simulink model "AN_Simulink_Model_v1_fil"  (R2019b)
settings: Solver=VariableStepAuto  StartTime=0.0  StopTime=testtime  RelTol=1e-3
InitFcn:
  | AN_InitFcn_Callback
StopFcn:
  | AN_StopFcn_Callback
values from neighbouring files (symbols this model uses):
  tdres = 1/Fs    (= 2.08333333333e-05)    [AN_Set_Model_Parameters.m]
libraries: hdlmdlgenlib x163, simulink x4, fillib x1, dspsrcs4 x1
(part 4 of 5)

== system AN_Simulink_Model_v1_fil/Auditory Nerve Model/C1 Chirp Filter/Get C1 Coefficients/Add7 ==
  In1 : Inport
  In2 : Inport  Port=2
  Add7 : Sum  OutDataTypeStr=single  SampleTime=2.08333333333333e-05  SaturateOnIntegerOverflow=on  InputSameDT=on
  Out1 : Outport
  wires:
  Add7/1 -> Out1/1
  In2/1 -> Add7/2
  In1/1 -> Add7/1

== system AN_Simulink_Model_v1_fil/Auditory Nerve Model/C1 Chirp Filter/Get C1 Coefficients/Add8 ==
  In1 : Inport
  In2 : Inport  Port=2
  Add8 : Sum  OutDataTypeStr=single  SampleTime=2.08333333333333e-05  SaturateOnIntegerOverflow=on  InputSameDT=on
  Out1 : Outport
  wires:
  Add8/1 -> Out1/1
  In2/1 -> Add8/2
  In1/1 -> Add8/1

== system AN_Simulink_Model_v1_fil/Auditory Nerve Model/C1 Chirp Filter/Get C1 Coefficients/Add9 ==
  In1 : Inport
  In2 : Inport  Port=2
  Add9 : Sum  OutDataTypeStr=single  SampleTime=2.08333333333333e-05  SaturateOnIntegerOverflow=on  InputSameDT=on
  Out1 : Outport
  wires:
  Add9/1 -> Out1/1
  In2/1 -> Add9/2
  In1/1 -> Add9/1

== system AN_Simulink_Model_v1_fil/Auditory Nerve Model/C1 Chirp Filter/Get C1 Coefficients/Divide1 ==
  In1 : Inport
  In2 : Inport  Port=2
  Divide1 : Product  Inputs=*/  OutDataTypeStr=single  SampleTime=2.08333333333333e-05  SaturateOnIntegerOverflow=on  RndMeth=Zero
  Out1 : Outport
  wires:
  Divide1/1 -> Out1/1
  In2/1 -> Divide1/2
  In1/1 -> Divide1/1

== system AN_Simulink_Model_v1_fil/Auditory Nerve Model/C1 Chirp Filter/Get C1 Coefficients/Divide10 ==
  In1 : Inport
  In2 : Inport  Port=2
  Divide10 : Product  Inputs=*/  OutDataTypeStr=single  SampleTime=2.08333333333333e-05  SaturateOnIntegerOverflow=on  RndMeth=Zero
  Out1 : Outport
  wires:
  Divide10/1 -> Out1/1
  In2/1 -> Divide10/2
  In1/1 -> Divide10/1

== system AN_Simulink_Model_v1_fil/Auditory Nerve Model/C1 Chirp Filter/Get C1 Coefficients/Divide11 ==
  In1 : Inport
  In2 : Inport  Port=2
  Divide11 : Product  Inputs=*/  OutDataTypeStr=single  SampleTime=2.08333333333333e-05  SaturateOnIntegerOverflow=on  RndMeth=Zero
  Out1 : Outport
  wires:
  Divide11/1 -> Out1/1
  In2/1 -> Divide11/2
  In1/1 -> Divide11/1

== system AN_Simulink_Model_v1_fil/Auditory Nerve Model/C1 Chirp Filter/Get C1 Coefficients/Divide12 ==
  In1 : Inport
  In2 : Inport  Port=2
  Divide12 : Product  Inputs=*/  OutDataTypeStr=single  SampleTime=2.08333333333333e-05  SaturateOnIntegerOverflow=on  RndMeth=Zero
  Out1 : Outport
  wires:
  Divide12/1 -> Out1/1
  In2/1 -> Divide12/2
  In1/1 -> Divide12/1

== system AN_Simulink_Model_v1_fil/Auditory Nerve Model/C1 Chirp Filter/Get C1 Coefficients/Divide13 ==
  In1 : Inport
  In2 : Inport  Port=2
  Divide13 : Product  Inputs=*/  OutDataTypeStr=single  SampleTime=2.08333333333333e-05  SaturateOnIntegerOverflow=on  RndMeth=Zero
  Out1 : Outport
  wires:
  Divide13/1 -> Out1/1
  In2/1 -> Divide13/2
  In1/1 -> Divide13/1

== system AN_Simulink_Model_v1_fil/Auditory Nerve Model/C1 Chirp Filter/Get C1 Coefficients/Divide14 ==
  In1 : Inport
  In2 : Inport  Port=2
  Divide14 : Product  Inputs=*/  OutDataTypeStr=single  SampleTime=2.08333333333333e-05  SaturateOnIntegerOverflow=on  RndMeth=Zero
  Out1 : Outport
  wires:
  Divide14/1 -> Out1/1
  In2/1 -> Divide14/2
  In1/1 -> Divide14/1

== system AN_Simulink_Model_v1_fil/Auditory Nerve Model/C1 Chirp Filter/Get C1 Coefficients/Divide15 ==
  In1 : Inport
  In2 : Inport  Port=2
  Divide15 : Product  Inputs=*/  OutDataTypeStr=single  SampleTime=2.08333333333333e-05  SaturateOnIntegerOverflow=on  RndMeth=Zero
  Out1 : Outport
  wires:
  Divide15/1 -> Out1/1
  In2/1 -> Divide15/2
  In1/1 -> Divide15/1

== system AN_Simulink_Model_v1_fil/Auditory Nerve Model/C1 Chirp Filter/Get C1 Coefficients/Divide16 ==
  In1 : Inport
  In2 : Inport  Port=2
  Divide16 : Product  Inputs=*/  OutDataTypeStr=single  SampleTime=2.08333333333333e-05  SaturateOnIntegerOverflow=on  RndMeth=Zero
  Out1 : Outport
  wires:
  Divide16/1 -> Out1/1
  In2/1 -> Divide16/2
  In1/1 -> Divide16/1

== system AN_Simulink_Model_v1_fil/Auditory Nerve Model/C1 Chirp Filter/Get C1 Coefficients/Divide17 ==
  In1 : Inport
  In2 : Inport  Port=2
  Divide17 : Product  Inputs=*/  OutDataTypeStr=single  SampleTime=2.08333333333333e-05  SaturateOnIntegerOverflow=on  RndMeth=Zero
  Out1 : Outport
  wires:
  Divide17/1 -> Out1/1
  In2/1 -> Divide17/2
  In1/1 -> Divide17/1

== system AN_Simulink_Model_v1_fil/Auditory Nerve Model/C1 Chirp Filter/Get C1 Coefficients/Divide18 ==
  In1 : Inport
  In2 : Inport  Port=2
  Divide18 : Product  Inputs=*/  OutDataTypeStr=single  SampleTime=2.08333333333333e-05  SaturateOnIntegerOverflow=on  RndMeth=Zero
  Out1 : Outport
  wires:
  Divide18/1 -> Out1/1
  In2/1 -> Divide18/2
  In1/1 -> Divide18/1

== system AN_Simulink_Model_v1_fil/Auditory Nerve Model/C1 Chirp Filter/Get C1 Coefficients/Divide19 ==
  In1 : Inport
  In2 : Inport  Port=2
  Divide19 : Product  Inputs=*/  OutDataTypeStr=single  SampleTime=2.08333333333333e-05  SaturateOnIntegerOverflow=on  RndMeth=Zero
  Out1 : Outport
  wires:
  Divide19/1 -> Out1/1
  In2/1 -> Divide19/2
  In1/1 -> Divide19/1

== system AN_Simulink_Model_v1_fil/Auditory Nerve Model/C1 Chirp Filter/Get C1 Coefficients/Divide2 ==
  In1 : Inport
  In2 : Inport  Port=2
  Divide2 : Product  Inputs=*/  OutDataTypeStr=single  SampleTime=2.08333333333333e-05  SaturateOnIntegerOverflow=on  RndMeth=Zero
  Out1 : Outport
  wires:
  Divide2/1 -> Out1/1
  In2/1 -> Divide2/2
  In1/1 -> Divide2/1

== system AN_Simulink_Model_v1_fil/Auditory Nerve Model/C1 Chirp Filter/Get C1 Coefficients/Divide20 ==
  In1 : Inport
  In2 : Inport  Port=2
  Divide20 : Product  Inputs=*/  OutDataTypeStr=single  SampleTime=2.08333333333333e-05  SaturateOnIntegerOverflow=on  RndMeth=Zero
  Out1 : Outport
  wires:
  Divide20/1 -> Out1/1
  In2/1 -> Divide20/2
  In1/1 -> Divide20/1

== system AN_Simulink_Model_v1_fil/Auditory Nerve Model/C1 Chirp Filter/Get C1 Coefficients/Divide21 ==
  In1 : Inport
  In2 : Inport  Port=2
  Divide21 : Product  Inputs=*/  OutDataTypeStr=single  SampleTime=2.08333333333333e-05  SaturateOnIntegerOverflow=on  RndMeth=Zero
  Out1 : Outport
  wires:
  Divide21/1 -> Out1/1
  In2/1 -> Divide21/2
  In1/1 -> Divide21/1

== system AN_Simulink_Model_v1_fil/Auditory Nerve Model/C1 Chirp Filter/Get C1 Coefficients/Divide22 ==
  In1 : Inport
  In2 : Inport  Port=2
  Divide22 : Product  Inputs=*/  OutDataTypeStr=single  SampleTime=2.08333333333333e-05  SaturateOnIntegerOverflow=on  RndMeth=Zero
  Out1 : Outport
  wires:
  Divide22/1 -> Out1/1
  In2/1 -> Divide22/2
  In1/1 -> Divide22/1

== system AN_Simulink_Model_v1_fil/Auditory Nerve Model/C1 Chirp Filter/Get C1 Coefficients/Divide23 ==
  In1 : Inport
  In2 : Inport  Port=2
  Divide23 : Product  Inputs=*/  OutDataTypeStr=single  SampleTime=2.08333333333333e-05  SaturateOnIntegerOverflow=on  RndMeth=Zero
  Out1 : Outport
  wires:
  Divide23/1 -> Out1/1
  In2/1 -> Divide23/2
  In1/1 -> Divide23/1

== system AN_Simulink_Model_v1_fil/Auditory Nerve Model/C1 Chirp Filter/Get C1 Coefficients/Divide3 ==
  In1 : Inport
  In2 : Inport  Port=2
  Divide3 : Product  Inputs=*/  OutDataTypeStr=single  SampleTime=2.08333333333333e-05  SaturateOnIntegerOverflow=on  RndMeth=Zero
  Out1 : Outport
  wires:
  Divide3/1 -> Out1/1
  In2/1 -> Divide3/2
  In1/1 -> Divide3/1

== system AN_Simulink_Model_v1_fil/Auditory Nerve Model/C1 Chirp Filter/Get C1 Coefficients/Divide4 ==
  In1 : Inport
  In2 : Inport  Port=2
  Divide4 : Product  Inputs=*/  OutDataTypeStr=single  SampleTime=2.08333333333333e-05  SaturateOnIntegerOverflow=on  RndMeth=Zero
  Out1 : Outport
  wires:
  Divide4/1 -> Out1/1
  In2/1 -> Divide4/2
  In1/1 -> Divide4/1

== system AN_Simulink_Model_v1_fil/Auditory Nerve Model/C1 Chirp Filter/Get C1 Coefficients/Divide5 ==
  In1 : Inport
  In2 : Inport  Port=2
  Divide5 : Product  Inputs=*/  OutDataTypeStr=single  SampleTime=2.08333333333333e-05  SaturateOnIntegerOverflow=on  RndMeth=Zero
  Out1 : Outport
  wires:
  Divide5/1 -> Out1/1
  In2/1 -> Divide5/2
  In1/1 -> Divide5/1

== system AN_Simulink_Model_v1_fil/Auditory Nerve Model/C1 Chirp Filter/Get C1 Coefficients/Divide6 ==
  In1 : Inport
  In2 : Inport  Port=2
  Divide6 : Product  Inputs=*/  OutDataTypeStr=single  SampleTime=2.08333333333333e-05  SaturateOnIntegerOverflow=on  RndMeth=Zero
  Out1 : Outport
  wires:
  Divide6/1 -> Out1/1
  In2/1 -> Divide6/2
  In1/1 -> Divide6/1

== system AN_Simulink_Model_v1_fil/Auditory Nerve Model/C1 Chirp Filter/Get C1 Coefficients/Divide7 ==
  In1 : Inport
  In2 : Inport  Port=2
  Divide7 : Product  Inputs=*/  OutDataTypeStr=single  SampleTime=2.08333333333333e-05  SaturateOnIntegerOverflow=on  RndMeth=Zero
  Out1 : Outport
  wires:
  Divide7/1 -> Out1/1
  In2/1 -> Divide7/2
  In1/1 -> Divide7/1

== system AN_Simulink_Model_v1_fil/Auditory Nerve Model/C1 Chirp Filter/Get C1 Coefficients/Divide8 ==
  In1 : Inport
  In2 : Inport  Port=2
  Divide8 : Product  Inputs=*/  OutDataTypeStr=single  SampleTime=2.08333333333333e-05  SaturateOnIntegerOverflow=on  RndMeth=Zero
  Out1 : Outport
  wires:
  Divide8/1 -> Out1/1
  In2/1 -> Divide8/2
  In1/1 -> Divide8/1

== system AN_Simulink_Model_v1_fil/Auditory Nerve Model/C1 Chirp Filter/Get C1 Coefficients/Divide9 ==
  In1 : Inport
  In2 : Inport  Port=2
  Divide9 : Product  Inputs=*/  OutDataTypeStr=single  SampleTime=2.08333333333333e-05  SaturateOnIntegerOverflow=on  RndMeth=Zero
  Out1 : Outport
  wires:
  Divide9/1 -> Out1/1
  In2/1 -> Divide9/2
  In1/1 -> Divide9/1

== system AN_Simulink_Model_v1_fil/Auditory Nerve Model/C1 Chirp Filter/Get C1 Coefficients/Gain10_unaryminus ==
  In1 : Inport
  Gain10_unaryminus : UnaryMinus  SampleTime=2.08333333333333e-05
  Out1 : Outport
  wires:
  Gain10_unaryminus/1 -> Out1/1
  In1/1 -> Gain10_unaryminus/1

== system AN_Simulink_Model_v1_fil/Auditory Nerve Model/C1 Chirp Filter/Get C1 Coefficients/Gain11 ==
  In1 : Inport
  Gain11 : Gain  Gain=single(2)
  Out1 : Outport
  wires:
  Gain11/1 -> Out1/1
  In1/1 -> Gain11/1

== system AN_Simulink_Model_v1_fil/Auditory Nerve Model/C1 Chirp Filter/Get C1 Coefficients/Gain12 ==
  In1 : Inport
  Gain12 : Gain  Gain=single(2)
  Out1 : Outport
  wires:
  Gain12/1 -> Out1/1
  In1/1 -> Gain12/1

== system AN_Simulink_Model_v1_fil/Auditory Nerve Model/C1 Chirp Filter/Get C1 Coefficients/Gain13 ==
  In1 : Inport
  Gain13 : Gain  Gain=single(2)
  Out1 : Outport
  wires:
  Gain13/1 -> Out1/1
  In1/1 -> Gain13/1

== system AN_Simulink_Model_v1_fil/Auditory Nerve Model/C1 Chirp Filter/Get C1 Coefficients/Gain14_unaryminus ==
  In1 : Inport
  Gain14_unaryminus : UnaryMinus  SampleTime=2.08333333333333e-05
  Out1 : Outport
  wires:
  Gain14_unaryminus/1 -> Out1/1
  In1/1 -> Gain14_unaryminus/1

== system AN_Simulink_Model_v1_fil/Auditory Nerve Model/C1 Chirp Filter/Get C1 Coefficients/Gain1_unaryminus ==
  In1 : Inport
  Gain1_unaryminus : UnaryMinus  SampleTime=2.08333333333333e-05
  Out1 : Outport
  wires:
  Gain1_unaryminus/1 -> Out1/1
  In1/1 -> Gain1_unaryminus/1

== system AN_Simulink_Model_v1_fil/Auditory Nerve Model/C1 Chirp Filter/Get C1 Coefficients/Gain2_unaryminus ==
  In1 : Inport
  Gain2_unaryminus : UnaryMinus  SampleTime=2.08333333333333e-05
  Out1 : Outport
  wires:
  Gain2_unaryminus/1 -> Out1/1
  In1/1 -> Gain2_unaryminus/1

== system AN_Simulink_Model_v1_fil/Auditory Nerve Model/C1 Chirp Filter/Get C1 Coefficients/Gain3_unaryminus ==
  In1 : Inport
  Gain3_unaryminus : UnaryMinus  SampleTime=2.08333333333333e-05
  Out1 : Outport
  wires:
  Gain3_unaryminus/1 -> Out1/1
  In1/1 -> Gain3_unaryminus/1

== system AN_Simulink_Model_v1_fil/Auditory Nerve Model/C1 Chirp Filter/Get C1 Coefficients/Gain4 ==
  In1 : Inport
  Gain4 : Gain  Gain=single(2)
  Out1 : Outport
  wires:
  Gain4/1 -> Out1/1
  In1/1 -> Gain4/1

== system AN_Simulink_Model_v1_fil/Auditory Nerve Model/C1 Chirp Filter/Get C1 Coefficients/Gain5 ==
  In1 : Inport
  Gain5 : Gain  Gain=single(2)
  Out1 : Outport
  wires:
  Gain5/1 -> Out1/1
  In1/1 -> Gain5/1

== system AN_Simulink_Model_v1_fil/Auditory Nerve Model/C1 Chirp Filter/Get C1 Coefficients/Gain6_unaryminus ==
  In1 : Inport
  Gain6_unaryminus : UnaryMinus  SampleTime=2.08333333333333e-05
  Out1 : Outport
  wires:
  Gain6_unaryminus/1 -> Out1/1
  In1/1 -> Gain6_unaryminus/1

== system AN_Simulink_Model_v1_fil/Auditory Nerve Model/C1 Chirp Filter/Get C1 Coefficients/Gain7 ==
  In1 : Inport
  Gain7 : Gain  Gain=single(-2)
  Out1 : Outport
  wires:
  Gain7/1 -> Out1/1
  In1/1 -> Gain7/1

== system AN_Simulink_Model_v1_fil/Auditory Nerve Model/C1 Chirp Filter/Get C1 Coefficients/Gain9_unaryminus ==
  In1 : Inport
  Gain9_unaryminus : UnaryMinus  SampleTime=2.08333333333333e-05
  Out1 : Outport
  wires:
  Gain9_unaryminus/1 -> Out1/1
  In1/1 -> Gain9_unaryminus/1

== system AN_Simulink_Model_v1_fil/Auditory Nerve Model/C1 Chirp Filter/Get C1 Coefficients/Product28 ==
  In1 : Inport
  In2 : Inport  Port=2
  Product28 : Product  Inputs=**  OutDataTypeStr=single  SampleTime=2.08333333333333e-05
  Out1 : Outport
  wires:
  Product28/1 -> Out1/1
  In2/1 -> Product28/2
  In1/1 -> Product28/1

== system AN_Simulink_Model_v1_fil/Auditory Nerve Model/C1 Chirp Filter/Get C1 Coefficients/Product29 ==
  In1 : Inport
  In2 : Inport  Port=2
  Product29 : Product  Inputs=**  OutDataTypeStr=single  SampleTime=2.08333333333333e-05
  Out1 : Outport
  wires:
  Product29/1 -> Out1/1
  In2/1 -> Product29/2
  In1/1 -> Product29/1

== system AN_Simulink_Model_v1_fil/Auditory Nerve Model/C1 Chirp Filter/Get C1 Coefficients/Product30 ==
  In1 : Inport
  In2 : Inport  Port=2
  Product30 : Product  Inputs=**  OutDataTypeStr=single  SampleTime=2.08333333333333e-05
  Out1 : Outport
  wires:
  Product30/1 -> Out1/1
  In2/1 -> Product30/2
  In1/1 -> Product30/1

== system AN_Simulink_Model_v1_fil/Auditory Nerve Model/C1 Chirp Filter/Get C1 Coefficients/Product34 ==
  In1 : Inport
  In2 : Inport  Port=2
  Product34 : Product  Inputs=**  OutDataTypeStr=single  SampleTime=2.08333333333333e-05
  Out1 : Outport
  wires:
  Product34/1 -> Out1/1
  In2/1 -> Product34/2
  In1/1 -> Product34/1

== system AN_Simulink_Model_v1_fil/Auditory Nerve Model/C1 Chirp Filter/Get C1 Coefficients/Product35 ==
  In1 : Inport
  In2 : Inport  Port=2
  Product35 : Product  Inputs=**  OutDataTypeStr=single  SampleTime=2.08333333333333e-05
  Out1 : Outport
  wires:
  Product35/1 -> Out1/1
  In2/1 -> Product35/2
  In1/1 -> Product35/1

== system AN_Simulink_Model_v1_fil/Auditory Nerve Model/C1 Chirp Filter/Get C1 Coefficients/Product36 ==
  In1 : Inport
  In2 : Inport  Port=2
  Product36 : Product  Inputs=**  OutDataTypeStr=single  SampleTime=2.08333333333333e-05
  Out1 : Outport
  wires:
  Product36/1 -> Out1/1
  In2/1 -> Product36/2
  In1/1 -> Product36/1

== system AN_Simulink_Model_v1_fil/Auditory Nerve Model/C1 Chirp Filter/Get C1 Coefficients/Product37 ==
  In1 : Inport
  In2 : Inport  Port=2
  Product37 : Product  Inputs=**  OutDataTypeStr=single  SampleTime=2.08333333333333e-05
  Out1 : Outport
  wires:
  Product37/1 -> Out1/1
  In2/1 -> Product37/2
  In1/1 -> Product37/1

== system AN_Simulink_Model_v1_fil/Auditory Nerve Model/C1 Chirp Filter/Get C1 Coefficients/Product38 ==
  In1 : Inport
  In2 : Inport  Port=2
  Product38 : Product  Inputs=**  OutDataTypeStr=single  SampleTime=2.08333333333333e-05
  Out1 : Outport
  wires:
  Product38/1 -> Out1/1
  In2/1 -> Product38/2
  In1/1 -> Product38/1

== system AN_Simulink_Model_v1_fil/Auditory Nerve Model/C1 Chirp Filter/Get C1 Coefficients/Product39 ==
  In1 : Inport
  In2 : Inport  Port=2
  Product39 : Product  Inputs=**  OutDataTypeStr=single  SampleTime=2.08333333333333e-05
  Out1 : Outport
  wires:
  Product39/1 -> Out1/1
  In2/1 -> Product39/2
  In1/1 -> Product39/1

== system AN_Simulink_Model_v1_fil/Auditory Nerve Model/C1 Chirp Filter/Get C1 Coefficients/Subtract ==
  In1 : Inport
  In2 : Inport  Port=2
  Subtract : Sum  Inputs=+-  OutDataTypeStr=single  SampleTime=2.08333333333333e-05  SaturateOnIntegerOverflow=on  InputSameDT=on
  Out1 : Outport
  wires:
  Subtract/1 -> Out1/1
  In2/1 -> Subtract/2
  In1/1 -> Subtract/1

== system AN_Simulink_Model_v1_fil/Auditory Nerve Model/C1 Chirp Filter/Get C1 Coefficients/Subtract1 ==
  In1 : Inport
  In2 : Inport  Port=2
  Subtract1 : Sum  Inputs=+-  OutDataTypeStr=single  SampleTime=2.08333333333333e-05  SaturateOnIntegerOverflow=on  InputSameDT=on
  Out1 : Outport
  wires:
  Subtract1/1 -> Out1/1
  In2/1 -> Subtract1/2
  In1/1 -> Subtract1/1

== system AN_Simulink_Model_v1_fil/Auditory Nerve Model/C1 Chirp Filter/Get C1 Coefficients/Subtract10 ==
  In1 : Inport
  In2 : Inport  Port=2
  Subtract10 : Sum  Inputs=+-  OutDataTypeStr=single  SampleTime=2.08333333333333e-05  SaturateOnIntegerOverflow=on  InputSameDT=on
  Out1 : Outport
  wires:
  Subtract10/1 -> Out1/1
  In2/1 -> Subtract10/2
  In1/1 -> Subtract10/1

== system AN_Simulink_Model_v1_fil/Auditory Nerve Model/C1 Chirp Filter/Get C1 Coefficients/Subtract11 ==
  In1 : Inport
  In2 : Inport  Port=2
  Subtract11 : Sum  Inputs=+-  OutDataTypeStr=single  SampleTime=2.08333333333333e-05  SaturateOnIntegerOverflow=on  InputSameDT=on
  Out1 : Outport
  wires:
  Subtract11/1 -> Out1/1
  In2/1 -> Subtract11/2
  In1/1 -> Subtract11/1

== system AN_Simulink_Model_v1_fil/Auditory Nerve Model/C1 Chirp Filter/Get C1 Coefficients/Subtract12 ==
  In1 : Inport
  In2 : Inport  Port=2
  Subtract12 : Sum  Inputs=+-  OutDataTypeStr=single  SampleTime=2.08333333333333e-05  SaturateOnIntegerOverflow=on  InputSameDT=on
  Out1 : Outport
  wires:
  Subtract12/1 -> Out1/1
  In2/1 -> Subtract12/2
  In1/1 -> Subtract12/1

== system AN_Simulink_Model_v1_fil/Auditory Nerve Model/C1 Chirp Filter/Get C1 Coefficients/Subtract13 ==
  In1 : Inport
  In2 : Inport  Port=2
  Subtract13 : Sum  Inputs=+-  OutDataTypeStr=single  SampleTime=2.08333333333333e-05  SaturateOnIntegerOverflow=on  InputSameDT=on
  Out1 : Outport
  wires:
  Subtract13/1 -> Out1/1
  In2/1 -> Subtract13/2
  In1/1 -> Subtract13/1

== system AN_Simulink_Model_v1_fil/Auditory Nerve Model/C1 Chirp Filter/Get C1 Coefficients/Subtract2 ==
  In1 : Inport
  In2 : Inport  Port=2
  Subtract2 : Sum  Inputs=+-  OutDataTypeStr=single  SampleTime=2.08333333333333e-05  SaturateOnIntegerOverflow=on  InputSameDT=on
  Out1 : Outport
  wires:
  Subtract2/1 -> Out1/1
  In2/1 -> Subtract2/2
  In1/1 -> Subtract2/1

== system AN_Simulink_Model_v1_fil/Auditory Nerve Model/C1 Chirp Filter/Get C1 Coefficients/Subtract6 ==
  In1 : Inport
  In2 : Inport  Port=2
  Subtract6 : Sum  Inputs=--  OutDataTypeStr=single  SampleTime=2.08333333333333e-05  SaturateOnIntegerOverflow=on  InputSameDT=on
  Out1 : Outport
  wires:
  Subtract6/1 -> Out1/1
  In2/1 -> Subtract6/2
  In1/1 -> Subtract6/1

== system AN_Simulink_Model_v1_fil/Auditory Nerve Model/C1 Chirp Filter/Get C1 Coefficients/Subtract7 ==
  In1 : Inport
  In2 : Inport  Port=2
  Subtract7 : Sum  Inputs=--  OutDataTypeStr=single  SampleTime=2.08333333333333e-05  SaturateOnIntegerOverflow=on  InputSameDT=on
  Out1 : Outport
  wires:
  Subtract7/1 -> Out1/1
  In2/1 -> Subtract7/2
  In1/1 -> Subtract7/1

== system AN_Simulink_Model_v1_fil/Auditory Nerve Model/C1 Chirp Filter/Get C1 Coefficients/Subtract8 ==
  In1 : Inport
  In2 : Inport  Port=2
  Subtract8 : Sum  Inputs=--  OutDataTypeStr=single  SampleTime=2.08333333333333e-05  SaturateOnIntegerOverflow=on  InputSameDT=on
  Out1 : Outport
  wires:
  Subtract8/1 -> Out1/1
  In2/1 -> Subtract8/2
  In1/1 -> Subtract8/1

== system AN_Simulink_Model_v1_fil/Auditory Nerve Model/C1 Chirp Filter/Get C1 Coefficients/Subtract9 ==
  In1 : Inport
  In2 : Inport  Port=2
  Subtract9 : Sum  Inputs=+-  OutDataTypeStr=single  SampleTime=2.08333333333333e-05  SaturateOnIntegerOverflow=on  InputSameDT=on
  Out1 : Outport
  wires:
  Subtract9/1 -> Out1/1
  In2/1 -> Subtract9/2
  In1/1 -> Subtract9/1

== system AN_Simulink_Model_v1_fil/Auditory Nerve Model/C1 Chirp Filter/Get C1 Coefficients/Trigonometric Function ==
  In1 : Inport
  Trigonometric Function : Trigonometry  Operator=atan  SampleTime=2.08333333333333e-05
  Out1 : Outport
  wires:
  Trigonometric Function/1 -> Out1/1
  In1/1 -> Trigonometric Function/1

== system AN_Simulink_Model_v1_fil/Auditory Nerve Model/C1 Chirp Filter/Get C1 Coefficients/Trigonometric Function1 ==
  In1 : Inport
  Trigonometric Function1 : Trigonometry  Operator=atan  SampleTime=2.08333333333333e-05
  Out1 : Outport
  wires:
  Trigonometric Function1/1 -> Out1/1
  In1/1 -> Trigonometric Function1/1

== system AN_Simulink_Model_v1_fil/Auditory Nerve Model/C1 Chirp Filter/Get C1 Coefficients/Trigonometric Function2 ==
  In1 : Inport
  Trigonometric Function2 : Trigonometry  Operator=atan  SampleTime=2.08333333333333e-05
  Out1 : Outport
  wires:
  Trigonometric Function2/1 -> Out1/1
  In1/1 -> Trigonometric Function2/1

== system AN_Simulink_Model_v1_fil/Auditory Nerve Model/C1 Chirp Filter/Get C1 Coefficients/Trigonometric Function3 ==
  In1 : Inport
  Trigonometric Function3 : Trigonometry  Operator=atan  SampleTime=2.08333333333333e-05
  Out1 : Outport
  wires:
  Trigonometric Function3/1 -> Out1/1
  In1/1 -> Trigonometric Function3/1

== system AN_Simulink_Model_v1_fil/Auditory Nerve Model/C1 Chirp Filter/Get C1 Coefficients/Trigonometric Function4 ==
  In1 : Inport
  Trigonometric Function4 : Trigonometry  Operator=atan  SampleTime=2.08333333333333e-05
  Out1 : Outport
  wires:
  Trigonometric Function4/1 -> Out1/1
  In1/1 -> Trigonometric Function4/1

== system AN_Simulink_Model_v1_fil/Auditory Nerve Model/C1 Chirp Filter/Get C1 Coefficients/Trigonometric Function5 ==
  In1 : Inport
  Trigonometric Function5 : Trigonometry  Operator=atan  SampleTime=2.08333333333333e-05
  Out1 : Outport
  wires:
  Trigonometric Function5/1 -> Out1/1
  In1/1 -> Trigonometric Function5/1

== system AN_Simulink_Model_v1_fil/Auditory Nerve Model/C1 Chirp Filter/Get C1 Coefficients/Trigonometric Function6 ==
  In1 : Inport
  Trigonometric Function6 : Trigonometry  Operator=tan  SampleTime=2.08333333333333e-05
  Out1 : Outport
  wires:
  Trigonometric Function6/1 -> Out1/1
  In1/1 -> Trigonometric Function6/1

== system AN_Simulink_Model_v1_fil/Auditory Nerve Model/C2 Wideband Filter/Calculate C2filterout/Abs ==
  In1 : Inport
  Abs : Abs  SampleTime=2.08333333333333e-05  OutDataTypeStr=single
  Out1 : Outport
  wires:
  Abs/1 -> Out1/1
  In1/1 -> Abs/1

== system AN_Simulink_Model_v1_fil/Auditory Nerve Model/C2 Wideband Filter/Calculate C2filterout/Divide ==
  In1 : Inport
  In2 : Inport  Port=2
  Divide : Product  Inputs=*/  OutDataTypeStr=single  SampleTime=2.08333333333333e-05  SaturateOnIntegerOverflow=on  RndMeth=Zero
  Out1 : Outport
  wires:
  Divide/1 -> Out1/1
  In2/1 -> Divide/2
  In1/1 -> Divide/1

== system AN_Simulink_Model_v1_fil/Auditory Nerve Model/C2 Wideband Filter/Calculate C2filterout/Divide1 ==
  In1 : Inport
  In2 : Inport  Port=2
  Divide1 : Product  Inputs=*/  OutDataTypeStr=single  SampleTime=2.08333333333333e-05  SaturateOnIntegerOverflow=on  RndMeth=Zero
  Out1 : Outport
  wires:
  Divide1/1 -> Out1/1
  In2/1 -> Divide1/2
  In1/1 -> Divide1/1

== system AN_Simulink_Model_v1_fil/Auditory Nerve Model/C2 Wideband Filter/Calculate C2filterout/Product ==
  In1 : Inport
  In2 : Inport  Port=2
  Product : Product  Inputs=**  OutDataTypeStr=single  SampleTime=2.08333333333333e-05
  Out1 : Outport
  wires:
  Product/1 -> Out1/1
  In2/1 -> Product/2
  In1/1 -> Product/1

== system AN_Simulink_Model_v1_fil/Auditory Nerve Model/C2 Wideband Filter/Calculate C2filterout/Product1 ==
  In1 : Inport
  In2 : Inport  Port=2
  Product1 : Product  Inputs=**  OutDataTypeStr=single  SampleTime=2.08333333333333e-05
  Out1 : Outport
  wires:
  Product1/1 -> Out1/1
  In2/1 -> Product1/2
  In1/1 -> Product1/1

== system AN_Simulink_Model_v1_fil/Auditory Nerve Model/C2 Wideband Filter/Calculate C2filterout/Product2 ==
  In1 : Inport
  In2 : Inport  Port=2
  Product2 : Product  Inputs=**  OutDataTypeStr=single  SampleTime=2.08333333333333e-05
  Out1 : Outport
  wires:
  Product2/1 -> Out1/1
  In2/1 -> Product2/2
  In1/1 -> Product2/1

== system AN_Simulink_Model_v1_fil/Auditory Nerve Model/Subsystem/IHC C1 NL Logarithmic Function/Abs1 ==
  In1 : Inport
  Abs1 : Abs  SampleTime=2.08333333333333e-05  OutDataTypeStr=single
  Out1 : Outport
  wires:
  Abs1/1 -> Out1/1
  In1/1 -> Abs1/1

== system AN_Simulink_Model_v1_fil/Auditory Nerve Model/Subsystem/IHC C1 NL Logarithmic Function/Add1 ==
  In1 : Inport
  In2 : Inport  Port=2
  Add1 : Sum  OutDataTypeStr=single  SampleTime=2.08333333333333e-05  SaturateOnIntegerOverflow=on  InputSameDT=on
  Out1 : Outport
  wires:
  Add1/1 -> Out1/1
  In2/1 -> Add1/2
  In1/1 -> Add1/1

== system AN_Simulink_Model_v1_fil/Auditory Nerve Model/Subsystem/IHC C1 NL Logarithmic Function/Compare To Zero1_relop ==
  In1 : Inport
  In2 : Inport  Port=2
  Compare To Zero1_relop : RelationalOperator  Operator=<  OutDataTypeStr=boolean  SampleTime=2.08333333333333e-05  RndMeth=Nearest  InputSameDT=on
  Out1 : Outport
  wires:
  Compare To Zero1_relop/1 -> Out1/1
  In2/1 -> Compare To Zero1_relop/2
  In1/1 -> Compare To Zero1_relop/1

== system AN_Simulink_Model_v1_fil/Auditory Nerve Model/Subsystem/IHC C1 NL Logarithmic Function/Log1 ==
  In1 : Inport
  Log1 : Math  Operator=log  SampleTime=2.08333333333333e-05  SaturateOnIntegerOverflow=on
  Out1 : Outport
  wires:
  Log1/1 -> Out1/1
  In1/1 -> Log1/1

== system AN_Simulink_Model_v1_fil/Auditory Nerve Model/Subsystem/IHC C1 NL Logarithmic Function/Product3 ==
  In1 : Inport
  In2 : Inport  Port=2
  Product3 : Product  Inputs=**  OutDataTypeStr=single  SampleTime=2.08333333333333e-05
  Out1 : Outport
  wires:
  Product3/1 -> Out1/1
  In2/1 -> Product3/2
  In1/1 -> Product3/1

== system AN_Simulink_Model_v1_fil/Auditory Nerve Model/Subsystem/IHC C1 NL Logarithmic Function/Product4 ==
  In1 : Inport
  In2 : Inport  Port=2
  Product4 : Product  Inputs=**  OutDataTypeStr=single  SampleTime=2.08333333333333e-05
  Out1 : Outport
  wires:
  Product4/1 -> Out1/1
  In2/1 -> Product4/2
  In1/1 -> Product4/1

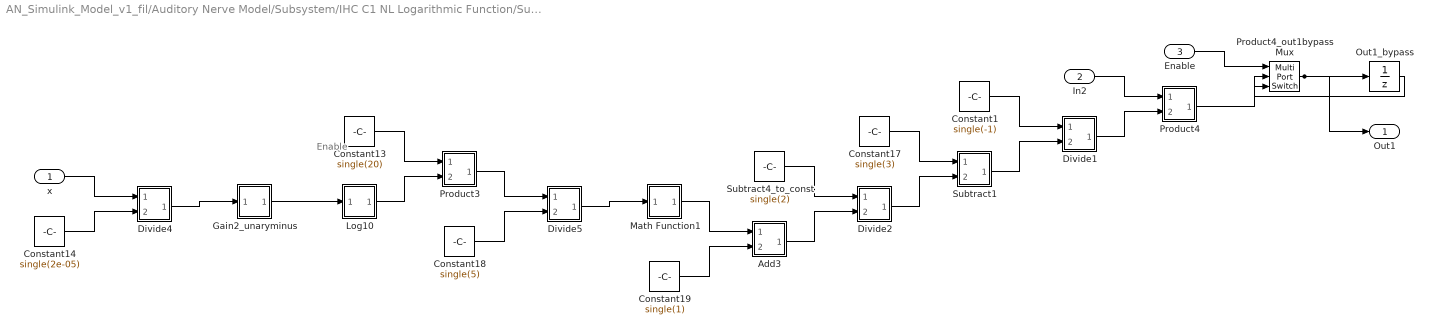
== system AN_Simulink_Model_v1_fil/Auditory Nerve Model/Subsystem/IHC C1 NL Logarithmic Function/Subsystem1 ==
  note: Enable
  x : Inport  OutDataTypeStr=single  PortDimensions=1  SampleTime=2.08333333333333e-05
  In2 : Inport  Port=2  OutDataTypeStr=single  PortDimensions=1  SampleTime=2.08333333333333e-05
  Enable : Inport  Port=3  OutDataTypeStr=boolean  SampleTime=2.08333333333333e-05
  Add3 : Subsystem
      mask Display: disp('NFP\nadd');
  Constant1 : Constant  Value=single(-1)  OutDataTypeStr=single  SampleTime=-1
  Constant13 : Constant  Value=single(20)  OutDataTypeStr=single  SampleTime=-1
  Constant14 : Constant  Value=single(2e-05)  OutDataTypeStr=single  SampleTime=-1
  Constant17 : Constant  Value=single(3)  OutDataTypeStr=single  SampleTime=-1
  Constant18 : Constant  Value=single(5)  OutDataTypeStr=single  SampleTime=-1
  Constant19 : Constant  Value=single(1)  OutDataTypeStr=single  SampleTime=-1
  Divide1 : Subsystem
      mask Display: disp('NFP\nmul');
  Divide2 : Subsystem
      mask Display: disp('NFP\nmul');
  Divide4 : Subsystem
      mask Display: disp('NFP\nmul');
  Divide5 : Subsystem
      mask Display: disp('NFP\nmul');
  Gain2_unaryminus : Subsystem
      mask Display: disp('NFP\numinus');
  Log10 : Subsystem
      mask Display: disp('NFP\nmath');
  Math Function1 : Subsystem
      mask Display: disp('NFP\nmath');
  Out1_bypass : UnitDelay  SampleTime=2.08333333333333e-05
  Product3 : Subsystem
      mask Display: disp('NFP\nmul');
  Product4 : Subsystem
      mask Display: disp('NFP\nmul');
  Product4_out1bypassMux : MultiPortSwitch  DataPortOrder=Zero-based contiguous  Inputs=2  zeroidx=on  OutDataTypeStr=single  SampleTime=2.08333333333333e-05
  Subtract1 : Subsystem
      mask Display: disp('NFP\nadd');
  Subtract4_to_const : Constant  Value=single(2)  OutDataTypeStr=single  SampleTime=-1
  Out1 : Outport  OutDataTypeStr=single  InitialOutput=0
  wires:
  Subtract1/1(Out1) -> Divide1/2(In2)
  Product4/1(Out1) -> Product4_out1bypassMux/3
  Product3/1(Out1) -> Divide5/1(In1)
  Math Function1/1(Out1) -> Add3/1(In1)
  Log10/1(Out1) -> Product3/2(In2)
  Divide5/1(Out1) -> Math Function1/1(In1)
  Divide4/1(Out1) -> Gain2_unaryminus/1(In1)
  Divide2/1(Out1) -> Subtract1/2(In2)
  Divide1/1(Out1) -> Product4/2(In2)
  Add3/1(Out1) -> Divide2/2(In2)
  Gain2_unaryminus/1(Out1) -> Log10/1(In1)
  Out1_bypass/1 -> Product4_out1bypassMux/2
  Product4_out1bypassMux/1 -> Out1/1, Out1_bypass/1
  Subtract4_to_const/1 -> Divide2/1(In1)
  Constant19/1 -> Add3/2(In2)
  Constant18/1 -> Divide5/2(In2)
  Constant17/1 -> Subtract1/1(In1)
  Constant14/1 -> Divide4/2(In2)
  Constant13/1 -> Product3/1(In1)
  Constant1/1 -> Divide1/1(In1)
  In2/1 -> Product4/1(In1)
  x/1 -> Divide4/1(In1)
  Enable/1 -> Product4_out1bypassMux/1

== system AN_Simulink_Model_v1_fil/Auditory Nerve Model/Subsystem/IHC C2 NL Logarithmic Function/Abs1 ==
  In1 : Inport
  Abs1 : Abs  SampleTime=2.08333333333333e-05  OutDataTypeStr=single
  Out1 : Outport
  wires:
  Abs1/1 -> Out1/1
  In1/1 -> Abs1/1

== system AN_Simulink_Model_v1_fil/Auditory Nerve Model/Subsystem/IHC C2 NL Logarithmic Function/Add1 ==
  In1 : Inport
  In2 : Inport  Port=2
  Add1 : Sum  OutDataTypeStr=single  SampleTime=2.08333333333333e-05  SaturateOnIntegerOverflow=on  InputSameDT=on
  Out1 : Outport
  wires:
  Add1/1 -> Out1/1
  In2/1 -> Add1/2
  In1/1 -> Add1/1

== system AN_Simulink_Model_v1_fil/Auditory Nerve Model/Subsystem/IHC C2 NL Logarithmic Function/Compare To Zero1_relop ==
  In1 : Inport
  In2 : Inport  Port=2
  Compare To Zero1_relop : RelationalOperator  Operator=<  OutDataTypeStr=boolean  SampleTime=2.08333333333333e-05  RndMeth=Nearest  InputSameDT=on
  Out1 : Outport
  wires:
  Compare To Zero1_relop/1 -> Out1/1
  In2/1 -> Compare To Zero1_relop/2
  In1/1 -> Compare To Zero1_relop/1

== system AN_Simulink_Model_v1_fil/Auditory Nerve Model/Subsystem/IHC C2 NL Logarithmic Function/Log1 ==
  In1 : Inport
  Log1 : Math  Operator=log  SampleTime=2.08333333333333e-05  SaturateOnIntegerOverflow=on
  Out1 : Outport
  wires:
  Log1/1 -> Out1/1
  In1/1 -> Log1/1

== system AN_Simulink_Model_v1_fil/Auditory Nerve Model/Subsystem/IHC C2 NL Logarithmic Function/Product3 ==
  In1 : Inport
  In2 : Inport  Port=2
  Product3 : Product  Inputs=**  OutDataTypeStr=single  SampleTime=2.08333333333333e-05
  Out1 : Outport
  wires:
  Product3/1 -> Out1/1
  In2/1 -> Product3/2
  In1/1 -> Product3/1

== system AN_Simulink_Model_v1_fil/Auditory Nerve Model/Subsystem/IHC C2 NL Logarithmic Function/Product4 ==
  In1 : Inport
  In2 : Inport  Port=2
  Product4 : Product  Inputs=**  OutDataTypeStr=single  SampleTime=2.08333333333333e-05
  Out1 : Outport
  wires:
  Product4/1 -> Out1/1
  In2/1 -> Product4/2
  In1/1 -> Product4/1

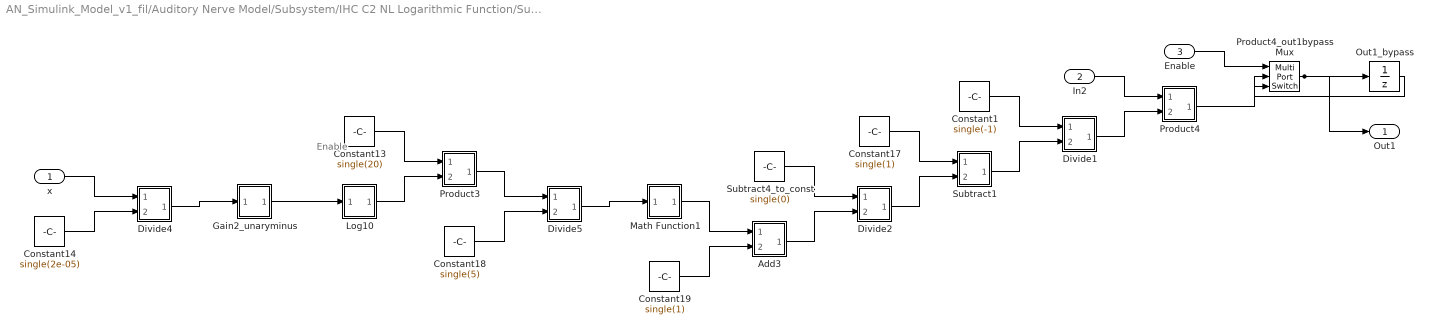
== system AN_Simulink_Model_v1_fil/Auditory Nerve Model/Subsystem/IHC C2 NL Logarithmic Function/Subsystem1 ==
  note: Enable
  x : Inport  OutDataTypeStr=single  PortDimensions=1  SampleTime=2.08333333333333e-05
  In2 : Inport  Port=2  OutDataTypeStr=single  PortDimensions=1  SampleTime=2.08333333333333e-05
  Enable : Inport  Port=3  OutDataTypeStr=boolean  SampleTime=2.08333333333333e-05
  Add3 : Subsystem
      mask Display: disp('NFP\nadd');
  Constant1 : Constant  Value=single(-1)  OutDataTypeStr=single  SampleTime=-1
  Constant13 : Constant  Value=single(20)  OutDataTypeStr=single  SampleTime=-1
  Constant14 : Constant  Value=single(2e-05)  OutDataTypeStr=single  SampleTime=-1
  Constant17 : Constant  Value=single(1)  OutDataTypeStr=single  SampleTime=-1
  Constant18 : Constant  Value=single(5)  OutDataTypeStr=single  SampleTime=-1
  Constant19 : Constant  Value=single(1)  OutDataTypeStr=single  SampleTime=-1
  Divide1 : Subsystem
      mask Display: disp('NFP\nmul');
  Divide2 : Subsystem
      mask Display: disp('NFP\nmul');
  Divide4 : Subsystem
      mask Display: disp('NFP\nmul');
  Divide5 : Subsystem
      mask Display: disp('NFP\nmul');
  Gain2_unaryminus : Subsystem
      mask Display: disp('NFP\numinus');
  Log10 : Subsystem
      mask Display: disp('NFP\nmath');
  Math Function1 : Subsystem
      mask Display: disp('NFP\nmath');
  Out1_bypass : UnitDelay  SampleTime=2.08333333333333e-05
  Product3 : Subsystem
      mask Display: disp('NFP\nmul');
  Product4 : Subsystem
      mask Display: disp('NFP\nmul');
  Product4_out1bypassMux : MultiPortSwitch  DataPortOrder=Zero-based contiguous  Inputs=2  zeroidx=on  OutDataTypeStr=single  SampleTime=2.08333333333333e-05
  Subtract1 : Subsystem
      mask Display: disp('NFP\nadd');
  Subtract4_to_const : Constant  Value=single(0)  OutDataTypeStr=single  SampleTime=-1
  Out1 : Outport  OutDataTypeStr=single  InitialOutput=0
  wires:
  Subtract1/1(Out1) -> Divide1/2(In2)
  Product4/1(Out1) -> Product4_out1bypassMux/3
  Product3/1(Out1) -> Divide5/1(In1)
  Math Function1/1(Out1) -> Add3/1(In1)
  Log10/1(Out1) -> Product3/2(In2)
  Divide5/1(Out1) -> Math Function1/1(In1)
  Divide4/1(Out1) -> Gain2_unaryminus/1(In1)
  Divide2/1(Out1) -> Subtract1/2(In2)
  Divide1/1(Out1) -> Product4/2(In2)
  Add3/1(Out1) -> Divide2/2(In2)
  Gain2_unaryminus/1(Out1) -> Log10/1(In1)
  Out1_bypass/1 -> Product4_out1bypassMux/2
  Product4_out1bypassMux/1 -> Out1/1, Out1_bypass/1
  Subtract4_to_const/1 -> Divide2/1(In1)
  Constant19/1 -> Add3/2(In2)
  Constant18/1 -> Divide5/2(In2)
  Constant17/1 -> Subtract1/1(In1)
  Constant14/1 -> Divide4/2(In2)
  Constant13/1 -> Product3/1(In1)
  Constant1/1 -> Divide1/1(In1)
  In2/1 -> Product4/1(In1)
  x/1 -> Divide4/1(In1)
  Enable/1 -> Product4_out1bypassMux/1

== system AN_Simulink_Model_v1_fil/Auditory Nerve Model/Subsystem/IHC LP Filter/Gain12_unaryminus ==
  In1 : Inport
  Gain12_unaryminus : UnaryMinus  SampleTime=2.08333333333333e-05
  Out1 : Outport
  wires:
  Gain12_unaryminus/1 -> Out1/1
  In1/1 -> Gain12_unaryminus/1

== system AN_Simulink_Model_v1_fil/Auditory Nerve Model/Subsystem/IHC LP Filter/Gain14_unaryminus ==
  In1 : Inport
  Gain14_unaryminus : UnaryMinus  SampleTime=2.08333333333333e-05
  Out1 : Outport
  wires:
  Gain14_unaryminus/1 -> Out1/1
  In1/1 -> Gain14_unaryminus/1

== system AN_Simulink_Model_v1_fil/Auditory Nerve Model/Subsystem/IHC LP Filter/Gain1_unaryminus ==
  In1 : Inport
  Gain1_unaryminus : UnaryMinus  SampleTime=2.08333333333333e-05
  Out1 : Outport
  wires:
  Gain1_unaryminus/1 -> Out1/1
  In1/1 -> Gain1_unaryminus/1

== system AN_Simulink_Model_v1_fil/Auditory Nerve Model/Subsystem/IHC LP Filter/Gain3_unaryminus ==
  In1 : Inport
  Gain3_unaryminus : UnaryMinus  SampleTime=2.08333333333333e-05
  Out1 : Outport
  wires:
  Gain3_unaryminus/1 -> Out1/1
  In1/1 -> Gain3_unaryminus/1

== system AN_Simulink_Model_v1_fil/Auditory Nerve Model/Subsystem/IHC LP Filter/Gain4_unaryminus ==
  In1 : Inport
  Gain4_unaryminus : UnaryMinus  SampleTime=2.08333333333333e-05
  Out1 : Outport
  wires:
  Gain4_unaryminus/1 -> Out1/1
  In1/1 -> Gain4_unaryminus/1

== system AN_Simulink_Model_v1_fil/Auditory Nerve Model/Subsystem/IHC LP Filter/Gain6_unaryminus ==
  In1 : Inport
  Gain6_unaryminus : UnaryMinus  SampleTime=2.08333333333333e-05
  Out1 : Outport
  wires:
  Gain6_unaryminus/1 -> Out1/1
  In1/1 -> Gain6_unaryminus/1

== system AN_Simulink_Model_v1_fil/Auditory Nerve Model/Subsystem/IHC LP Filter/Gain9_unaryminus ==
  In1 : Inport
  Gain9_unaryminus : UnaryMinus  SampleTime=2.08333333333333e-05
  Out1 : Outport
  wires:
  Gain9_unaryminus/1 -> Out1/1
  In1/1 -> Gain9_unaryminus/1

== system AN_Simulink_Model_v1_fil/Auditory Nerve Model/Subsystem/IHC LP Filter/Product12 ==
  In1 : Inport
  In2 : Inport  Port=2
  Product12 : Product  Inputs=**  OutDataTypeStr=single  SampleTime=2.08333333333333e-05
  Out1 : Outport
  wires:
  Product12/1 -> Out1/1
  In2/1 -> Product12/2
  In1/1 -> Product12/1

== system AN_Simulink_Model_v1_fil/Auditory Nerve Model/Subsystem/IHC LP Filter/Product13 ==
  In1 : Inport
  In2 : Inport  Port=2
  Product13 : Product  Inputs=**  OutDataTypeStr=single  SampleTime=2.08333333333333e-05
  Out1 : Outport
  wires:
  Product13/1 -> Out1/1
  In2/1 -> Product13/2
  In1/1 -> Product13/1

== system AN_Simulink_Model_v1_fil/Auditory Nerve Model/Subsystem/IHC LP Filter/Product14 ==
  In1 : Inport
  In2 : Inport  Port=2
  Product14 : Product  Inputs=**  OutDataTypeStr=single  SampleTime=2.08333333333333e-05
  Out1 : Outport
  wires:
  Product14/1 -> Out1/1
  In2/1 -> Product14/2
  In1/1 -> Product14/1

== system AN_Simulink_Model_v1_fil/Auditory Nerve Model/Subsystem/IHC LP Filter/Product17 ==
  In1 : Inport
  In2 : Inport  Port=2
  Product17 : Product  Inputs=**  OutDataTypeStr=single  SampleTime=2.08333333333333e-05
  Out1 : Outport
  wires:
  Product17/1 -> Out1/1
  In2/1 -> Product17/2
  In1/1 -> Product17/1

== system AN_Simulink_Model_v1_fil/Auditory Nerve Model/Subsystem/IHC LP Filter/Product18 ==
  In1 : Inport
  In2 : Inport  Port=2
  Product18 : Product  Inputs=**  OutDataTypeStr=single  SampleTime=2.08333333333333e-05
  Out1 : Outport
  wires:
  Product18/1 -> Out1/1
  In2/1 -> Product18/2
  In1/1 -> Product18/1

== system AN_Simulink_Model_v1_fil/Auditory Nerve Model/Subsystem/IHC LP Filter/Product19 ==
  In1 : Inport
  In2 : Inport  Port=2
  Product19 : Product  Inputs=**  OutDataTypeStr=single  SampleTime=2.08333333333333e-05
  Out1 : Outport
  wires:
  Product19/1 -> Out1/1
  In2/1 -> Product19/2
  In1/1 -> Product19/1

== system AN_Simulink_Model_v1_fil/Auditory Nerve Model/Subsystem/IHC LP Filter/Product2 ==
  In1 : Inport
  In2 : Inport  Port=2
  Product2 : Product  Inputs=**  OutDataTypeStr=single  SampleTime=2.08333333333333e-05
  Out1 : Outport
  wires:
  Product2/1 -> Out1/1
  In2/1 -> Product2/2
  In1/1 -> Product2/1

== system AN_Simulink_Model_v1_fil/Auditory Nerve Model/Subsystem/IHC LP Filter/Product22 ==
  In1 : Inport
  In2 : Inport  Port=2
  Product22 : Product  Inputs=**  OutDataTypeStr=single  SampleTime=2.08333333333333e-05
  Out1 : Outport
  wires:
  Product22/1 -> Out1/1
  In2/1 -> Product22/2
  In1/1 -> Product22/1

== system AN_Simulink_Model_v1_fil/Auditory Nerve Model/Subsystem/IHC LP Filter/Product23 ==
  In1 : Inport
  In2 : Inport  Port=2
  Product23 : Product  Inputs=**  OutDataTypeStr=single  SampleTime=2.08333333333333e-05
  Out1 : Outport
  wires:
  Product23/1 -> Out1/1
  In2/1 -> Product23/2
  In1/1 -> Product23/1

== system AN_Simulink_Model_v1_fil/Auditory Nerve Model/Subsystem/IHC LP Filter/Product24 ==
  In1 : Inport
  In2 : Inport  Port=2
  Product24 : Product  Inputs=**  OutDataTypeStr=single  SampleTime=2.08333333333333e-05
  Out1 : Outport
  wires:
  Product24/1 -> Out1/1
  In2/1 -> Product24/2
  In1/1 -> Product24/1

== system AN_Simulink_Model_v1_fil/Auditory Nerve Model/Subsystem/IHC LP Filter/Product27 ==
  In1 : Inport
  In2 : Inport  Port=2
  Product27 : Product  Inputs=**  OutDataTypeStr=single  SampleTime=2.08333333333333e-05
  Out1 : Outport
  wires:
  Product27/1 -> Out1/1
  In2/1 -> Product27/2
  In1/1 -> Product27/1

== system AN_Simulink_Model_v1_fil/Auditory Nerve Model/Subsystem/IHC LP Filter/Product28 ==
  In1 : Inport
  In2 : Inport  Port=2
  Product28 : Product  Inputs=**  OutDataTypeStr=single  SampleTime=2.08333333333333e-05
  Out1 : Outport
  wires:
  Product28/1 -> Out1/1
  In2/1 -> Product28/2
  In1/1 -> Product28/1

== system AN_Simulink_Model_v1_fil/Auditory Nerve Model/Subsystem/IHC LP Filter/Product29 ==
  In1 : Inport
  In2 : Inport  Port=2
  Product29 : Product  Inputs=**  OutDataTypeStr=single  SampleTime=2.08333333333333e-05
  Out1 : Outport
  wires:
  Product29/1 -> Out1/1
  In2/1 -> Product29/2
  In1/1 -> Product29/1

== system AN_Simulink_Model_v1_fil/Auditory Nerve Model/Subsystem/IHC LP Filter/Product3 ==
  In1 : Inport
  In2 : Inport  Port=2
  Product3 : Product  Inputs=**  OutDataTypeStr=single  SampleTime=2.08333333333333e-05
  Out1 : Outport
  wires:
  Product3/1 -> Out1/1
  In2/1 -> Product3/2
  In1/1 -> Product3/1

== system AN_Simulink_Model_v1_fil/Auditory Nerve Model/Subsystem/IHC LP Filter/Product32 ==
  In1 : Inport
  In2 : Inport  Port=2
  Product32 : Product  Inputs=**  OutDataTypeStr=single  SampleTime=2.08333333333333e-05
  Out1 : Outport
  wires:
  Product32/1 -> Out1/1
  In2/1 -> Product32/2
  In1/1 -> Product32/1

== system AN_Simulink_Model_v1_fil/Auditory Nerve Model/Subsystem/IHC LP Filter/Product33 ==
  In1 : Inport
  In2 : Inport  Port=2
  Product33 : Product  Inputs=**  OutDataTypeStr=single  SampleTime=2.08333333333333e-05
  Out1 : Outport
  wires:
  Product33/1 -> Out1/1
  In2/1 -> Product33/2
  In1/1 -> Product33/1

== system AN_Simulink_Model_v1_fil/Auditory Nerve Model/Subsystem/IHC LP Filter/Product34 ==
  In1 : Inport
  In2 : Inport  Port=2
  Product34 : Product  Inputs=**  OutDataTypeStr=single  SampleTime=2.08333333333333e-05
  Out1 : Outport
  wires:
  Product34/1 -> Out1/1
  In2/1 -> Product34/2
  In1/1 -> Product34/1

== system AN_Simulink_Model_v1_fil/Auditory Nerve Model/Subsystem/IHC LP Filter/Product4 ==
  In1 : Inport
  In2 : Inport  Port=2
  Product4 : Product  Inputs=**  OutDataTypeStr=single  SampleTime=2.08333333333333e-05
  Out1 : Outport
  wires:
  Product4/1 -> Out1/1
  In2/1 -> Product4/2
  In1/1 -> Product4/1

== system AN_Simulink_Model_v1_fil/Auditory Nerve Model/Subsystem/IHC LP Filter/Product7 ==
  In1 : Inport
  In2 : Inport  Port=2
  Product7 : Product  Inputs=**  OutDataTypeStr=single  SampleTime=2.08333333333333e-05
  Out1 : Outport
  wires:
  Product7/1 -> Out1/1
  In2/1 -> Product7/2
  In1/1 -> Product7/1

== system AN_Simulink_Model_v1_fil/Auditory Nerve Model/Subsystem/IHC LP Filter/Product8 ==
  In1 : Inport
  In2 : Inport  Port=2
  Product8 : Product  Inputs=**  OutDataTypeStr=single  SampleTime=2.08333333333333e-05
  Out1 : Outport
  wires:
  Product8/1 -> Out1/1
  In2/1 -> Product8/2
  In1/1 -> Product8/1

== system AN_Simulink_Model_v1_fil/Auditory Nerve Model/Subsystem/IHC LP Filter/Product9 ==
  In1 : Inport
  In2 : Inport  Port=2
  Product9 : Product  Inputs=**  OutDataTypeStr=single  SampleTime=2.08333333333333e-05
  Out1 : Outport
  wires:
  Product9/1 -> Out1/1
  In2/1 -> Product9/2
  In1/1 -> Product9/1

== system AN_Simulink_Model_v1_fil/Auditory Nerve Model/Subsystem/IHC LP Filter/Sum10 ==
  In1 : Inport
  In2 : Inport  Port=2
  Sum10 : Sum  OutDataTypeStr=single  SampleTime=2.08333333333333e-05  SaturateOnIntegerOverflow=on  InputSameDT=on
  Out1 : Outport
  wires:
  Sum10/1 -> Out1/1
  In2/1 -> Sum10/2
  In1/1 -> Sum10/1

== system AN_Simulink_Model_v1_fil/Auditory Nerve Model/Subsystem/IHC LP Filter/Sum11 ==
  In1 : Inport
  In2 : Inport  Port=2
  Sum11 : Sum  OutDataTypeStr=single  SampleTime=2.08333333333333e-05  SaturateOnIntegerOverflow=on  InputSameDT=on
  Out1 : Outport
  wires:
  Sum11/1 -> Out1/1
  In2/1 -> Sum11/2
  In1/1 -> Sum11/1

== system AN_Simulink_Model_v1_fil/Auditory Nerve Model/Subsystem/IHC LP Filter/Sum12 ==
  In1 : Inport
  In2 : Inport  Port=2
  Sum12 : Sum  OutDataTypeStr=single  SampleTime=2.08333333333333e-05  SaturateOnIntegerOverflow=on  InputSameDT=on
  Out1 : Outport
  wires:
  Sum12/1 -> Out1/1
  In2/1 -> Sum12/2
  In1/1 -> Sum12/1

== system AN_Simulink_Model_v1_fil/Auditory Nerve Model/Subsystem/IHC LP Filter/Sum13 ==
  In1 : Inport
  In2 : Inport  Port=2
  Sum13 : Sum  OutDataTypeStr=single  SampleTime=2.08333333333333e-05  SaturateOnIntegerOverflow=on  InputSameDT=on
  Out1 : Outport
  wires:
  Sum13/1 -> Out1/1
  In2/1 -> Sum13/2
  In1/1 -> Sum13/1

== system AN_Simulink_Model_v1_fil/Auditory Nerve Model/Subsystem/IHC LP Filter/Sum16 ==
  In1 : Inport
  In2 : Inport  Port=2
  Sum16 : Sum  OutDataTypeStr=single  SampleTime=2.08333333333333e-05  SaturateOnIntegerOverflow=on  InputSameDT=on
  Out1 : Outport
  wires:
  Sum16/1 -> Out1/1
  In2/1 -> Sum16/2
  In1/1 -> Sum16/1

== system AN_Simulink_Model_v1_fil/Auditory Nerve Model/Subsystem/IHC LP Filter/Sum17 ==
  In1 : Inport
  In2 : Inport  Port=2
  Sum17 : Sum  OutDataTypeStr=single  SampleTime=2.08333333333333e-05  SaturateOnIntegerOverflow=on  InputSameDT=on
  Out1 : Outport
  wires:
  Sum17/1 -> Out1/1
  In2/1 -> Sum17/2
  In1/1 -> Sum17/1

== system AN_Simulink_Model_v1_fil/Auditory Nerve Model/Subsystem/IHC LP Filter/Sum2 ==
  In1 : Inport
  In2 : Inport  Port=2
  Sum2 : Sum  OutDataTypeStr=single  SampleTime=2.08333333333333e-05  SaturateOnIntegerOverflow=on  InputSameDT=on
  Out1 : Outport
  wires:
  Sum2/1 -> Out1/1
  In2/1 -> Sum2/2
  In1/1 -> Sum2/1

== system AN_Simulink_Model_v1_fil/Auditory Nerve Model/Subsystem/IHC LP Filter/Sum20 ==
  In1 : Inport
  In2 : Inport  Port=2
  Sum20 : Sum  OutDataTypeStr=single  SampleTime=2.08333333333333e-05  SaturateOnIntegerOverflow=on  InputSameDT=on
  Out1 : Outport
  wires:
  Sum20/1 -> Out1/1
  In2/1 -> Sum20/2
  In1/1 -> Sum20/1

== system AN_Simulink_Model_v1_fil/Auditory Nerve Model/Subsystem/IHC LP Filter/Sum21 ==
  In1 : Inport
  In2 : Inport  Port=2
  Sum21 : Sum  OutDataTypeStr=single  SampleTime=2.08333333333333e-05  SaturateOnIntegerOverflow=on  InputSameDT=on
  Out1 : Outport
  wires:
  Sum21/1 -> Out1/1
  In2/1 -> Sum21/2
  In1/1 -> Sum21/1

== system AN_Simulink_Model_v1_fil/Auditory Nerve Model/Subsystem/IHC LP Filter/Sum24 ==
  In1 : Inport
  In2 : Inport  Port=2
  Sum24 : Sum  OutDataTypeStr=single  SampleTime=2.08333333333333e-05  SaturateOnIntegerOverflow=on  InputSameDT=on
  Out1 : Outport
  wires:
  Sum24/1 -> Out1/1
  In2/1 -> Sum24/2
  In1/1 -> Sum24/1

== system AN_Simulink_Model_v1_fil/Auditory Nerve Model/Subsystem/IHC LP Filter/Sum25 ==
  In1 : Inport
  In2 : Inport  Port=2
  Sum25 : Sum  OutDataTypeStr=single  SampleTime=2.08333333333333e-05  SaturateOnIntegerOverflow=on  InputSameDT=on
  Out1 : Outport
  wires:
  Sum25/1 -> Out1/1
  In2/1 -> Sum25/2
  In1/1 -> Sum25/1

== system AN_Simulink_Model_v1_fil/Auditory Nerve Model/Subsystem/IHC LP Filter/Sum3 ==
  In1 : Inport
  In2 : Inport  Port=2
  Sum3 : Sum  OutDataTypeStr=single  SampleTime=2.08333333333333e-05  SaturateOnIntegerOverflow=on  InputSameDT=on
  Out1 : Outport
  wires:
  Sum3/1 -> Out1/1
  In2/1 -> Sum3/2
  In1/1 -> Sum3/1

== system AN_Simulink_Model_v1_fil/Auditory Nerve Model/Subsystem/IHC LP Filter/Sum6 ==
  In1 : Inport
  In2 : Inport  Port=2
  Sum6 : Sum  OutDataTypeStr=single  SampleTime=2.08333333333333e-05  SaturateOnIntegerOverflow=on  InputSameDT=on
  Out1 : Outport
  wires:
  Sum6/1 -> Out1/1
  In2/1 -> Sum6/2
  In1/1 -> Sum6/1

== system AN_Simulink_Model_v1_fil/Auditory Nerve Model/Subsystem/IHC LP Filter/Sum7 ==
  In1 : Inport
  In2 : Inport  Port=2
  Sum7 : Sum  OutDataTypeStr=single  SampleTime=2.08333333333333e-05  SaturateOnIntegerOverflow=on  InputSameDT=on
  Out1 : Outport
  wires:
  Sum7/1 -> Out1/1
  In2/1 -> Sum7/2
  In1/1 -> Sum7/1

== system AN_Simulink_Model_v1_fil/Auditory Nerve Model/Subsystem/IHC C1 NL Logarithmic Function/Subsystem1/Add3 ==
  In1 : Inport
  In2 : Inport  Port=2
  Add3 : Sum  OutDataTypeStr=single  SampleTime=2.08333333333333e-05  SaturateOnIntegerOverflow=on  InputSameDT=on
  Out1 : Outport
  wires:
  Add3/1 -> Out1/1
  In2/1 -> Add3/2
  In1/1 -> Add3/1

== system AN_Simulink_Model_v1_fil/Auditory Nerve Model/Subsystem/IHC C1 NL Logarithmic Function/Subsystem1/Divide1 ==
  In1 : Inport
  In2 : Inport  Port=2
  Divide1 : Product  Inputs=*/  OutDataTypeStr=single  SampleTime=2.08333333333333e-05  SaturateOnIntegerOverflow=on  RndMeth=Zero
  Out1 : Outport
  wires:
  Divide1/1 -> Out1/1
  In2/1 -> Divide1/2
  In1/1 -> Divide1/1

== system AN_Simulink_Model_v1_fil/Auditory Nerve Model/Subsystem/IHC C1 NL Logarithmic Function/Subsystem1/Divide2 ==
  In1 : Inport
  In2 : Inport  Port=2
  Divide2 : Product  Inputs=*/  OutDataTypeStr=single  SampleTime=2.08333333333333e-05  SaturateOnIntegerOverflow=on  RndMeth=Zero
  Out1 : Outport
  wires:
  Divide2/1 -> Out1/1
  In2/1 -> Divide2/2
  In1/1 -> Divide2/1

== system AN_Simulink_Model_v1_fil/Auditory Nerve Model/Subsystem/IHC C1 NL Logarithmic Function/Subsystem1/Divide4 ==
  In1 : Inport
  In2 : Inport  Port=2
  Divide4 : Product  Inputs=*/  OutDataTypeStr=single  SampleTime=2.08333333333333e-05  SaturateOnIntegerOverflow=on  RndMeth=Zero
  Out1 : Outport
  wires:
  Divide4/1 -> Out1/1
  In2/1 -> Divide4/2
  In1/1 -> Divide4/1

== system AN_Simulink_Model_v1_fil/Auditory Nerve Model/Subsystem/IHC C1 NL Logarithmic Function/Subsystem1/Divide5 ==
  In1 : Inport
  In2 : Inport  Port=2
  Divide5 : Product  Inputs=*/  OutDataTypeStr=single  SampleTime=2.08333333333333e-05  SaturateOnIntegerOverflow=on  RndMeth=Zero
  Out1 : Outport
  wires:
  Divide5/1 -> Out1/1
  In2/1 -> Divide5/2
  In1/1 -> Divide5/1

== system AN_Simulink_Model_v1_fil/Auditory Nerve Model/Subsystem/IHC C1 NL Logarithmic Function/Subsystem1/Gain2_unaryminus ==
  In1 : Inport
  Gain2_unaryminus : UnaryMinus  SampleTime=2.08333333333333e-05
  Out1 : Outport
  wires:
  Gain2_unaryminus/1 -> Out1/1
  In1/1 -> Gain2_unaryminus/1

== system AN_Simulink_Model_v1_fil/Auditory Nerve Model/Subsystem/IHC C1 NL Logarithmic Function/Subsystem1/Log10 ==
  In1 : Inport
  Log10 : Math  Operator=log10  SampleTime=2.08333333333333e-05  SaturateOnIntegerOverflow=on
  Out1 : Outport
  wires:
  Log10/1 -> Out1/1
  In1/1 -> Log10/1

== system AN_Simulink_Model_v1_fil/Auditory Nerve Model/Subsystem/IHC C1 NL Logarithmic Function/Subsystem1/Math Function1 ==
  In1 : Inport
  Math Function1 : Math  SampleTime=2.08333333333333e-05  SaturateOnIntegerOverflow=on
  Out1 : Outport
  wires:
  Math Function1/1 -> Out1/1
  In1/1 -> Math Function1/1
